simulink model "shifter_matlab"  (R2018a)
settings: Solver=FixedStepDiscrete  StartTime=0.0  StopTime=30  FixedStep=0.05  RelTol=1e-3  EnableMultiTasking=on
PreLoadFcn:
  | load shifter_data;
settings Model: Creator=jrivitus  LastModifiedBy=bneiswan
settings DataIOCC: ExternalInput=[t, up_threshold, vehicle_speed, down_threshold]  LimitDataPoints=on  LoadExternalInput=on  SaveFormat=Array
settings OptimizationCC: ExpressionDepthLimit=2147483647  LifeSpan=inf
settings DebuggingCC: UnderspecifiedInitializationDetection=Classic  MergeDetectMultiDrivingBlocksExec=none  ParameterPrecisionLossMsg=none  FcnCallInpInsideContextMsg=warning  AllowSymbolicDim=off  StateNameClashWarn=warning  SFUnexpectedBacktrackingDiag=warning  SFNoUnconditionalDefaultTransitionDiag=warning  SFExecutionAtInitializationDiag=none
settings HardwareCC: ProdBitPerPointer=32  ProdBitPerSizeT=32  ProdBitPerPtrDiffT=32  ProdLargestAtomicFloat=None  ProdIntDivRoundTo=Undefined  ProdEndianess=Unspecified  ProdWordSize=32  ProdHWDeviceType=32-bit Generic
settings ModelReferenceCC: PropagateSignalLabelsOutOfModel=off
settings CodeAppCC: StateflowObjectComments=on
settings GRTTargetCC: TargetLangStandard=C89/C90 (ANSI)  GeneratePreprocessorConditionals=Disable all  CombineOutputUpdateFcns=off  GRTInterface=on
settings ConfigComp: CovMetricSettings=dw  CovHtmlReporting=on  CovSaveCumulativeToWorkspaceVar=on  CovSaveSingleToWorkspaceVar=on  CovExternalEMLEnable=off  CovSFcnEnable=off

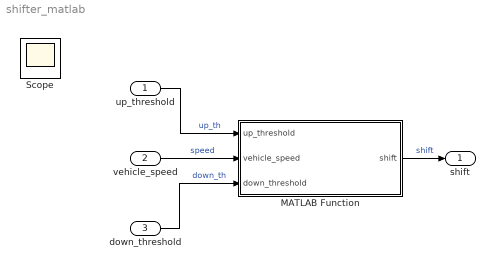
== system shifter_matlab ==
  up_threshold : Inport  OutDataTypeStr=double
  vehicle_speed : Inport  Port=2  OutDataTypeStr=double
  down_threshold : Inport  Port=3  OutDataTypeStr=double
  MATLAB Function : MATLAB Function  TreatAsAtomicUnit=on
  shift : Outport
  Scope : Scope
  wires:
  MATLAB Function/1(shift) -> shift/1  "shift"
  up_threshold/1 -> MATLAB Function/1(up_threshold)  "up_th"
  vehicle_speed/1 -> MATLAB Function/2(vehicle_speed)  "speed"
  down_threshold/1 -> MATLAB Function/3(down_threshold)  "down_th"

== matlab function shifter_matlab/MATLAB Function ==
  data: up_threshold input; shift output; vehicle_speed input; down_threshold input
function shift = fcn(up_threshold, vehicle_speed, down_threshold)
%#codegen

if (vehicle_speed > up_threshold)
    shift = 1;
elseif (vehicle_speed < down_threshold)
    shift = -1;
else
    shift = 0;
end
